simulink model "cartracker2"  (Simulink 6.4)
settings: Solver=FixedStepDiscrete  StartTime=0.0  StopTime=inf  RelTol=1e-3
InitFcn:
  | model_path = [regexprep(gcs, '/.*$', '') '/Edit Parameters'];
  | line_row = str2num(get_param(model_path,'line_row'));
  | min_area  = str2num(get_param(model_path,'min_area'));
  | max_area = str2num(get_param(model_path,'max_area'));
undefined symbols (not defined in the file or in its folder): Rec, SDTV, strel
libraries: dspmtrx3 x7, vipsnks x4, simulink x3, viptextngfix x3, vipmisc x2, vipconversions x2, vipmorphops x1, vipstatistics x1, dspindex x1, dspwin32 x1
CloseFcn:
  | clear line_row;
settings Model: Creator=don  LastModifiedBy=Raza  ExtModeAutoUpdateStatusClock=off
settings DataIOCC: LimitDataPoints=off  SaveOutput=off  SignalLogging=off  SaveTime=off  SignalLoggingName=sigsOut
settings OptimizationCC: BufferReusableBoundary=off
settings DebuggingCC: AlgebraicLoopMsg=none  CheckExecutionContextPreStartOutputMsg=on  CheckExecutionContextRuntimeOutputMsg=on  SolverPrmCheckMsg=none  ParameterPrecisionLossMsg=none  BusObjectLabelMismatch=none  StrictBusMsg=None
settings HardwareCC: TargetHWDeviceType=32-bit Generic  ProdEqTarget=off

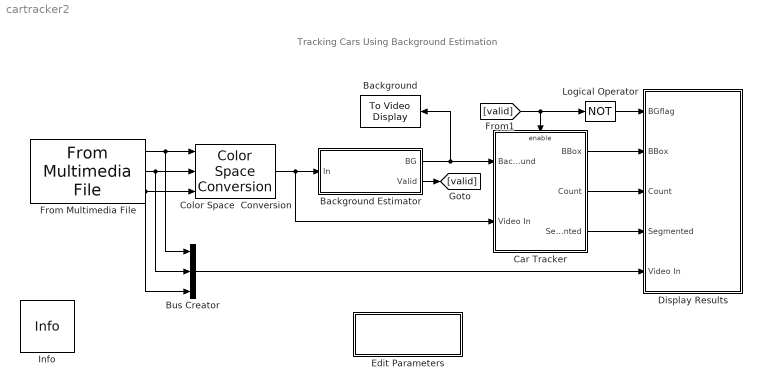
== system cartracker2 ==
  note: Tracking Cars Using Background Estimation
  Background : vipsnks/To Video Display  Orientation=left  inputType=Intensity  OutputDevice=On-screen video monitor  fullScreen=off  videoWindowX=372  videoWindowY=101  saveWindowSize=off  videoWindowWidth=168  videoWindowHeight=147
  Background Estimator : Subsystem  BlockChoice=Temporal Median Estimator
      settings: AttributesFormatString=%<BlockChoice>  MemberBlocks=Motion Based Background Estimator,Temporal Median,Temporal Median Estimator
      settings: TemplateBlock=|
      | vipmisc/Background
      | Estimator
  Bus Creator : BusCreator  Inputs=3
  Car Tracker : Subsystem  TreatAsAtomicUnit=on
  Color Space  Conversion : vipconversions/Color Space  Conversion  conversion=R'G'B' to intensity  wp_str=D65  rec=Rec. 601 (SDTV)  sys=1125/60/2:1
  Display Results : Subsystem
  Edit Parameters : Subsystem  mask(Edit Parameters){line_row=22, min_area=200, max_area=2500, BGEstimator=Estimating median over time}
      mask prompts: line_row "White line position (row):"; min_area "Minimum object area:"; max_area "Maximum object area:"; BGEstimator "Background estimation based on:"
      mask help: Modify model initialization parameters.
      mask init:
      | blk = [gcs '/Background Estimator'];
      | if BGEstimator == 1
      |     set_param(blk, 'BlockChoice', 'Temporal Median Estimator');
      | elseif BGEstimator == 2
      |     set_param(blk, 'BlockChoice', 'Temporal Median');
      | else
      |     set_param(blk, 'BlockChoice', 'Motion Based Background Estimator');
      | end
      mask StyleString: edit,edit,edit,popup(Estimating median over time|Computing median over time|Eliminating moving objects)
      mask Display: disp('Edit\nParameters')
  From Multimedia File : dspwin32/From Multimedia File  DialogController=dspDDGCreate  DialogControllerArgs=DataTag3  inputFilename=D:\Stuff\Study Material\FYP\whiz\MVI_1730.AVI  loop=on  numPlays=inf  outputStreams=Video only  videoDataType=single  audioDataType=int16  inheritSampleTime=on  userDefinedSampleTime=1/40  noAudioOutput=off  isIntensityVideo=off  outputEOF=off
  Info : vipmisc/Info  SystemSampleTime=-1
  Logical Operator : Logic  Operator=NOT  AllPortsSameDT=off  OutDataTypeMode=Boolean
  wires:
  From Multimedia File/1 -> Color Space  Conversion/1, Bus Creator/1
  From Multimedia File/2 -> Color Space  Conversion/2, Bus Creator/2
  From Multimedia File/3 -> Color Space  Conversion/3, Bus Creator/3
  Background Estimator/1(BG) -> Car Tracker/1(Background), Background/1
  Logical Operator/1 -> Display Results/1(BGflag)
  Bus Creator/1 -> Display Results/5(Video In)
  Car Tracker/1(BBox) -> Display Results/2(BBox)
  Car Tracker/2(Count) -> Display Results/3(Count)
  Car Tracker/3(Segmented) -> Display Results/4(Segmented)
  Color Space  Conversion/1 -> Car Tracker/2(Video In), Background Estimator/1(In)
  Background Estimator/2(Valid) -> [valid]
  [valid] -> Car Tracker/Enable, Logical Operator/1

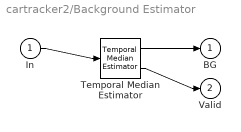
== system cartracker2/Background Estimator ==
  In : Inport
  Temporal Median Estimator : vipmisc/Temporal Median Estimator  SystemSampleTime=-1  t0=2
  BG : Outport
  Valid : Outport  Port=2
  wires:
  In/1 -> Temporal Median Estimator/1
  Temporal Median Estimator/1 -> BG/1
  Temporal Median Estimator/2 -> Valid/1

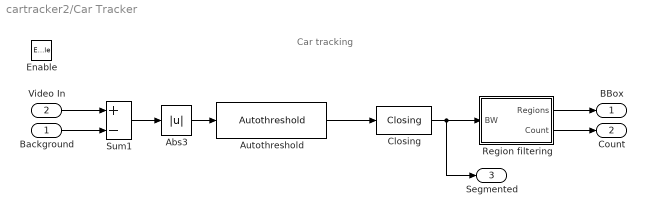
== system cartracker2/Car Tracker ==
  note: Car tracking
  Background : Inport
  Video In : Inport  Port=2
  Enable : EnablePort
  Abs3 : Abs  SaturateOnIntegerOverflow=on  SampleTime=-1
  Autothreshold : vipconversions/Autothreshold  DialogController=vipDDGCreate  DialogControllerArgs=DataTag0  operator=>  threshOut=off  effMetricOut=off  userDefinedRange=off  umin=0  umax=255  outOfRngOpt=Warn and saturate  scaleThreshold=off  scaleFactor=1  P1Mode=Specify word length  P1WordLength=32  P1FracLength=30  P2Mode=Specify word length  P2WordLength=32  P2FracLength=22  P3Mode=Specify word length  P3WordLength=32  P3FracLength=14  P4Mode=Binary point scaling  P4WordLength=32  P4FracLength=15  Q1Mode=Specify word length  Q1WordLength=32  Q1FracLength=16  EMMode=Specify word length  EMWordLength=16  EMFracLength=14  roundingMode=Floor  overflowMode=off
  Closing : vipmorphops/Closing  nhoodsrc=Specify via dialog  strel=strel('square',5)
  Region filtering : Subsystem
  Sum1 : Sum  Inputs=+-  SaturateOnIntegerOverflow=on  InputSameDT=on
  BBox : Outport
  Count : Outport  Port=2
  Segmented : Outport  Port=3
  wires:
  Video In/1 -> Sum1/1
  Background/1 -> Sum1/2
  Closing/1 -> Region filtering/1(BW), Segmented/1
  Abs3/1 -> Autothreshold/1
  Region filtering/1(Regions) -> BBox/1
  Autothreshold/1 -> Closing/1
  Sum1/1 -> Abs3/1
  Region filtering/2(Count) -> Count/1

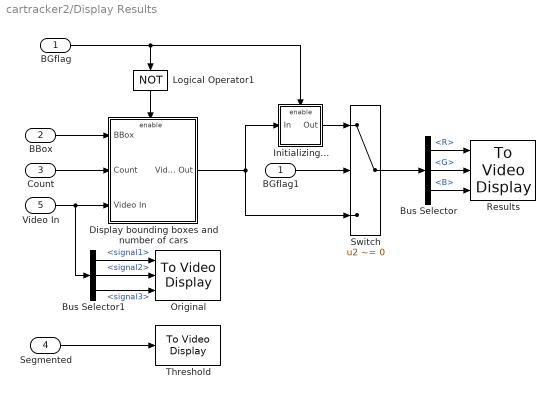
== system cartracker2/Display Results ==
  BGflag : Inport
  BBox : Inport  Port=2
  Count : Inport  Port=3
  Segmented : Inport  Port=4
  Video In : Inport  Port=5
  BGflag1 : InportShadow  Port=1  LatchByCopyingInsideSignal=off
  Bus Selector : BusSelector  OutputSignals=R,G,B
  Bus Selector1 : BusSelector  OutputSignals=signal1,signal2,signal3
  Display bounding boxes and number of cars : Subsystem
  Initializing... : Subsystem
  Logical Operator1 : Logic  Orientation=down  Operator=NOT
  Original : vipsnks/To Video Display  inputType=RGB  OutputDevice=On-screen video monitor  fullScreen=off  videoWindowX=196  videoWindowY=101  saveWindowSize=off  videoWindowWidth=168  videoWindowHeight=147
  Results : vipsnks/To Video Display  inputType=RGB  OutputDevice=On-screen video monitor  fullScreen=off  videoWindowX=720  videoWindowY=101  saveWindowSize=off  videoWindowWidth=168  videoWindowHeight=147
  Switch : Switch  Criteria=u2 ~= 0  Threshold=boolean(0)
  Threshold : vipsnks/To Video Display  inputType=Intensity  OutputDevice=On-screen video monitor  fullScreen=off  videoWindowX=544  videoWindowY=101  saveWindowSize=off  videoWindowWidth=168  videoWindowHeight=147
  wires:
  BGflag1/1 -> Switch/2
  BBox/1 -> Display bounding boxes and number of cars/1(BBox)
  Initializing.../1(Out) -> Switch/1
  Segmented/1 -> Threshold/1
  Display bounding boxes and number of cars/1(Video Out) -> Initializing.../1(In), Switch/3
  Count/1 -> Display bounding boxes and number of cars/2(Count)
  BGflag/1 -> Initializing.../Enable, Logical Operator1/1
  Logical Operator1/1 -> Display bounding boxes and number of cars/Enable
  Switch/1 -> Bus Selector/1
  Video In/1 -> Display bounding boxes and number of cars/3(Video In), Bus Selector1/1
  Bus Selector/1 -> Results/1  "<R>"
  Bus Selector/2 -> Results/2  "<G>"
  Bus Selector/3 -> Results/3  "<B>"
  Bus Selector1/1 -> Original/1  "<signal1>"
  Bus Selector1/2 -> Original/2  "<signal2>"
  Bus Selector1/3 -> Original/3  "<signal3>"

== system cartracker2/Edit Parameters ==

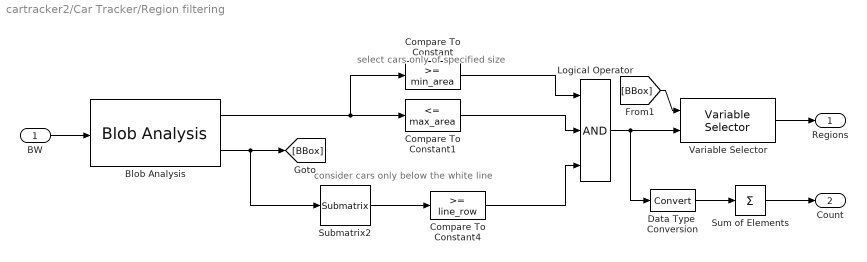
== system cartracker2/Car Tracker/Region filtering ==
  note: select cars only of specified size
  note: consider cars only below the white line
  BW : Inport
  Blob Analysis : vipstatistics/Blob Analysis  DialogController=vipDDGCreate  DialogControllerArgs=DataTag1  area=on  centroid=off  bBox=on  majorAxis=off  minorAxis=off  angle=off  eccentricity=off  equivDiameterSq=off  extent=off  perimeter=off  maxBlobs=80  warnIfNumBlobsExceeded=on  isCount=off  useMinArea=off  minArea=0  useMaxArea=off  maxArea=inf  excludeBorderBlob=off  outDT=double  isFill=on  fillValues=-1  conn=8  isLabel=off  outputMode=Binary point scaling  outputWordLength=32  outputFracLength=16  firstCoeffMode=Binary point scaling  firstCoeffWordLength=16  firstCoeffFracLength=14  secondCoeffMode=Binary point scaling  secondCoeffWordLength=32  secondCoeffFracLength=16  accumMode=Binary point scaling  accumWordLength=32  accumFracLength=0  prodOutputMode=Binary point scaling  prodOutputWordLength=32  prodOutputFracLength=16  roundingMode=Floor  overflowMode=off
  Compare To Constant : simulink/Logic and Bit Operations/Compare To Constant  SystemSampleTime=-1  relop=>=  const=min_area  LogicOutDataTypeMode=boolean  ZeroCross=off
  Compare To Constant1 : simulink/Logic and Bit Operations/Compare To Constant  SystemSampleTime=-1  relop=<=  const=max_area  LogicOutDataTypeMode=boolean  ZeroCross=off
  Compare To Constant4 : simulink/Logic and Bit Operations/Compare To Constant  SystemSampleTime=-1  relop=>=  const=line_row  LogicOutDataTypeMode=uint8  ZeroCross=off
  Data Type  Conversion : DataTypeConversion  OutDataTypeMode=uint8  SaturateOnIntegerOverflow=on  RndMeth=Zero
  Logical Operator : Logic  Inputs=3  AllPortsSameDT=off  OutDataTypeMode=Boolean
  Submatrix2 : dspmtrx3/Submatrix  RowSpan=One row  RowStartMode=Index  RowStartIndex=1  RowEndMode=Last  RowEndIndex=1  ColSpan=All columns  ColStartMode=First  ColStartIndex=1  ColEndMode=Last  ColEndIndex=1
  Sum of Elements : Sum  Inputs=+  OutScaling=2^-10
  Variable Selector : dspindex/Variable Selector  NumInputs=1  rowsOrCols=Columns  IdxMode=Variable  Elements=[1 3]  ZerOneIdxMode=Zero-based  errmode=Clip Index  FillMode=on  FillValues=-1
  Regions : Outport
  Count : Outport  Port=2
  wires:
  BW/1 -> Blob Analysis/1
  Blob Analysis/2 -> [BBox], Submatrix2/1
  Logical Operator/1 -> Variable Selector/2, Data Type  Conversion/1
  Compare To Constant/1 -> Logical Operator/1
  Compare To Constant1/1 -> Logical Operator/2
  Variable Selector/1 -> Regions/1
  Blob Analysis/1 -> Compare To Constant1/1, Compare To Constant/1
  [BBox] -> Variable Selector/1
  Submatrix2/1 -> Compare To Constant4/1
  Compare To Constant4/1 -> Logical Operator/3
  Sum of Elements/1 -> Count/1
  Data Type  Conversion/1 -> Sum of Elements/1

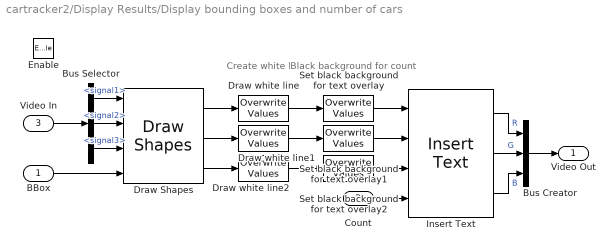
== system cartracker2/Display Results/Display bounding boxes and number of cars ==
  note: Create white
      | line
  note: Black background
      | for count
  BBox : Inport
  Count : Inport  Port=2
  Video In : Inport  Port=3
  Enable : EnablePort
  Bus Creator : BusCreator  Inputs=3
  Bus Selector : BusSelector  OutputSignals=signal1,signal2,signal3
  Draw Shapes : viptextngfix/Draw Shapes  DialogController=vipDDGCreate  DialogControllerArgs=DataTag2  inType=RGB  shape=Rectangles  fill=off  display=User-specified value  intensity=200  color=[0 1 0]  opacity=0.6  viewport=Entire image  antialiasing=off
  Draw white line : dspmtrx3/Overwrite Values  OverWriteDiag=Submatrix  valFrom2ndIP=Specify via dialog  ConstValue=1  RowSpan=Range of rows  RowStartMode=Index  RowStartIndex=line_row  RowEndMode=Index  RowEndIndex=line_row+1  ColSpan=All columns  ColStartMode=First  ColStartIndex=1  ColEndMode=Last  ColEndIndex=1  DiagSpan=Range of elements  DiagStartMode=Index  DiagStartIndex=2  DiagEndMode=Index  DiagEndIndex=4
  Draw white line1 : dspmtrx3/Overwrite Values  OverWriteDiag=Submatrix  valFrom2ndIP=Specify via dialog  ConstValue=1  RowSpan=Range of rows  RowStartMode=Index  RowStartIndex=line_row  RowEndMode=Index  RowEndIndex=line_row+1  ColSpan=All columns  ColStartMode=First  ColStartIndex=1  ColEndMode=Last  ColEndIndex=1  DiagSpan=Range of elements  DiagStartMode=Index  DiagStartIndex=2  DiagEndMode=Index  DiagEndIndex=4
  Draw white line2 : dspmtrx3/Overwrite Values  OverWriteDiag=Submatrix  valFrom2ndIP=Specify via dialog  ConstValue=1  RowSpan=Range of rows  RowStartMode=Index  RowStartIndex=line_row  RowEndMode=Index  RowEndIndex=line_row+1  ColSpan=All columns  ColStartMode=First  ColStartIndex=1  ColEndMode=Last  ColEndIndex=1  DiagSpan=Range of elements  DiagStartMode=Index  DiagStartIndex=2  DiagEndMode=Index  DiagEndIndex=4
  Insert Text : viptextngfix/Insert Text  inputType=RGB  theText='%4d'  fontFace=Arial  dummyVar1=0  blockFontSize=12  antiAliased=on  getTextLocFrom=Specify via dialog  textLoc=[0 0]  getTextColorFrom=Specify via dialog  textColor=[1 1 1]  getTextIntensityFrom=Specify via dialog  textIntensity=1  getTextOpacityFrom=Specify via dialog  textOpacity=1.0  dummyVar2=0  dummyVar3=0  dummyVar4=0
  Set black background for text overlay : dspmtrx3/Overwrite Values  OverWriteDiag=Submatrix  valFrom2ndIP=Specify via dialog  ConstValue=0  RowSpan=Range of rows  RowStartMode=First  RowStartIndex=25  RowEndMode=Index  RowEndIndex=15  ColSpan=Range of columns  ColStartMode=First  ColStartIndex=1  ColEndMode=Index  ColEndIndex=30  DiagSpan=Range of elements  DiagStartMode=Index  DiagStartIndex=2  DiagEndMode=Index  DiagEndIndex=4
  Set black background for text overlay1 : dspmtrx3/Overwrite Values  OverWriteDiag=Submatrix  valFrom2ndIP=Specify via dialog  ConstValue=0  RowSpan=Range of rows  RowStartMode=First  RowStartIndex=25  RowEndMode=Index  RowEndIndex=15  ColSpan=Range of columns  ColStartMode=First  ColStartIndex=1  ColEndMode=Index  ColEndIndex=30  DiagSpan=Range of elements  DiagStartMode=Index  DiagStartIndex=2  DiagEndMode=Index  DiagEndIndex=4
  Set black background for text overlay2 : dspmtrx3/Overwrite Values  OverWriteDiag=Submatrix  valFrom2ndIP=Specify via dialog  ConstValue=0  RowSpan=Range of rows  RowStartMode=First  RowStartIndex=25  RowEndMode=Index  RowEndIndex=15  ColSpan=Range of columns  ColStartMode=First  ColStartIndex=1  ColEndMode=Index  ColEndIndex=30  DiagSpan=Range of elements  DiagStartMode=Index  DiagStartIndex=2  DiagEndMode=Index  DiagEndIndex=4
  Video Out : Outport
  wires:
  Set black background for text overlay/1 -> Insert Text/1
  Draw white line/1 -> Set black background for text overlay/1
  Draw Shapes/1 -> Draw white line/1
  BBox/1 -> Draw Shapes/4
  Video In/1 -> Bus Selector/1
  Bus Selector/1 -> Draw Shapes/1  "<signal1>"
  Bus Selector/2 -> Draw Shapes/2  "<signal2>"
  Bus Selector/3 -> Draw Shapes/3  "<signal3>"
  Count/1 -> Insert Text/4
  Draw white line1/1 -> Set black background for text overlay1/1
  Draw white line2/1 -> Set black background for text overlay2/1
  Draw Shapes/2 -> Draw white line1/1
  Draw Shapes/3 -> Draw white line2/1
  Set black background for text overlay1/1 -> Insert Text/2
  Set black background for text overlay2/1 -> Insert Text/3
  Insert Text/1 -> Bus Creator/1  "R"
  Insert Text/2 -> Bus Creator/2  "G"
  Insert Text/3 -> Bus Creator/3  "B"
  Bus Creator/1 -> Video Out/1

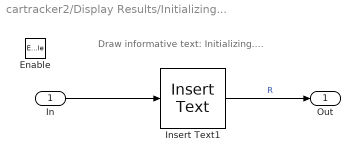
== system cartracker2/Display Results/Initializing... ==
  note: Draw informative text: Initializing....
  In : Inport
  Enable : EnablePort
  Insert Text1 : viptextngfix/Insert Text  inputType=Intensity  theText="'       initialization ...'"  fontFace=Arial  dummyVar1=0  blockFontSize=18  antiAliased=on  getTextLocFrom=Specify via dialog  textLoc=[0 0]  getTextColorFrom=Specify via dialog  textColor=[1 1 1]  getTextIntensityFrom=Specify via dialog  textIntensity=1  getTextOpacityFrom=Specify via dialog  textOpacity=1.0  dummyVar2=0  dummyVar3=0  dummyVar4=0
  Out : Outport
  wires:
  In/1 -> Insert Text1/1
  Insert Text1/1 -> Out/1  "R"
